simulink model "simulink_caso3_adc"  (R2023a)
settings: Solver=VariableStepAuto  StartTime=0.0  StopTime=10.0  RelTol=1e-3
undefined symbols (not defined in the file): A, Aestd, B, Bestd, C, Cestd, D, Destd, K00d, Ts
libraries: simulink x1
settings Model: Creator=Agustin  LastModifiedBy=Agustin

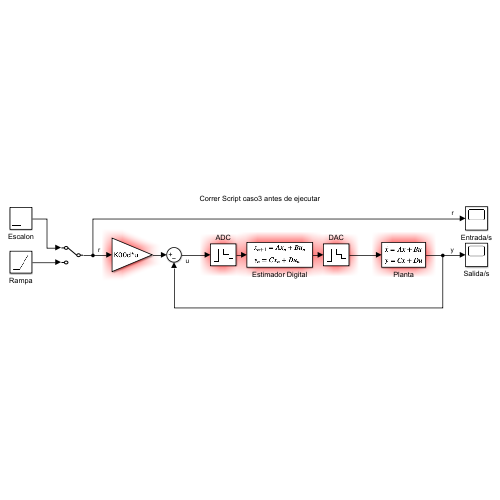
[thumbnail: Simulink's stored preview of the top-level diagram]
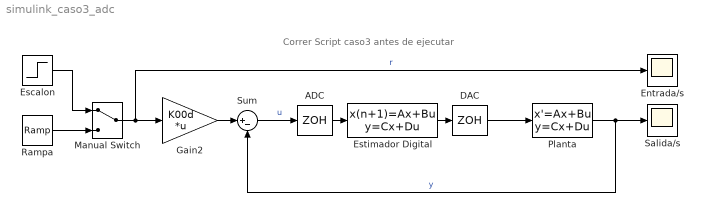
== system simulink_caso3_adc ==
  note: Correr Script caso3 antes de ejecutar
  ADC : ZeroOrderHold  SampleTime=Ts
  DAC : ZeroOrderHold  SampleTime=Ts
  Entrada/s : Scope
  Escalon : Step  SampleTime=0
  Estimador Digital : DiscreteStateSpace  A=Aestd  B=Bestd  C=Cestd  D=Destd  SampleTime=Ts
  Gain2 : Gain  Gain=K00d  Multiplication=Matrix(K*u)
  Manual Switch : ManualSwitch
  Planta : StateSpace  A=A  B=B  C=C  D=D  InitialCondition=0
  Rampa : simulink/Sources/Ramp  slope=1  start=0  InitialOutput=0
  Salida/s : Scope
  Sum : Sum  Inputs=|+-
  wires:
  Escalon/1 -> Manual Switch/1
  Estimador Digital/1 -> DAC/1
  Sum/1 -> ADC/1  "u"
  Rampa/1 -> Manual Switch/2
  Planta/1 -> Salida/s/1, Sum/2  "y"
  Manual Switch/1 -> Entrada/s/1, Gain2/1  "r"
  Gain2/1 -> Sum/1
  ADC/1 -> Estimador Digital/1
  DAC/1 -> Planta/1
